simulink model "DinsatHW7"  (R2021b)
settings: Solver=ode45  StartTime=0.0  StopTime=900  RelTol=1e-3
undefined symbols (not defined in the file): IAU
libraries: slpidlib x6, simulink_extras x3, aerolibtransform2 x2, vrlib x1
settings Model: PacingRate=1000  Creator=hilmi  LastModifiedBy=hilmi

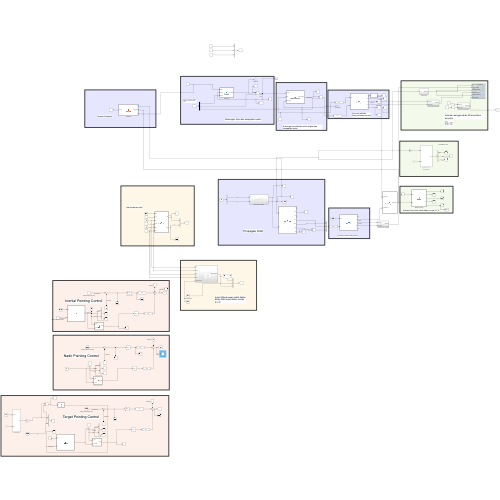
[thumbnail: Simulink's stored preview of the top-level diagram]
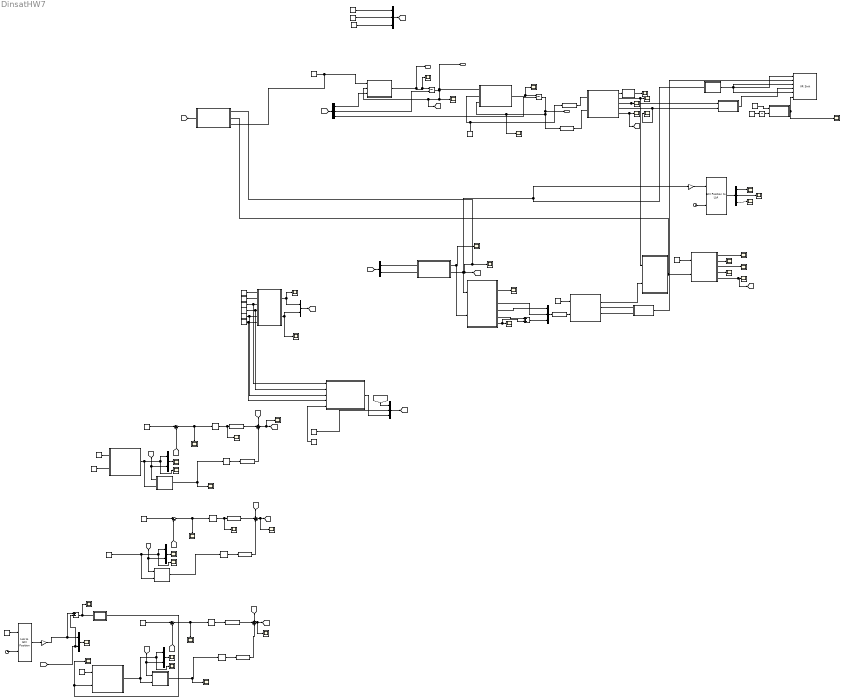
== system DinsatHW7 ==
  note: Gravity Gradient
  note: Inertial Pointing Control
  note: Input elemen orbit
  note: Koordinat LLA
  note: Attitude Body-Orbit satelit dalam urutan Z-Y-X
  note: Input Attitude awal satelit dalam
      | Body-Orbit input dalam urutan
      | Z-Y-X
  note: Koordinat orbit terhadap inersial
  note: Propagasi Orbit
  note: Input Torsi dan initial condition
      | tergantung keperluan setiap
      | nomor.
  note: notes:
      | Sumbu x+ : Merah
      | Sumbu y+ : Biru
      | Sumbu z+ : Hijau
  note: Animasi menggunakan 3D simulation simulink
  note: Konversi attitude
      | Body terhadap inersial
  note: Hubungan perubahan euler angles dan kecepatan sudut
  note: Hubungan torsi dan kecepatan sudut
  note: Nadir Pointing Control
  note: Target Pointing Control
  Add : Sum
  Add1 : Sum  Inputs=+-
  Attitude Body Orbit : MATLAB Function  TreatAsAtomicUnit=on
  BodyOrbit attitude input : Constant  Value=[30,20,30]
  Clock : Clock
  Clock1 : Clock
  Constant{,1,5,25} (4 alike) : Constant  Value=[3,2,1]
  Constant15 : Constant  Value=6903
  Constant19 : Constant  Value=0
  Constant2 : Constant  Value=[1,0,0,0]
  Constant20 : Constant  Value=1e-5
  Constant21 : Constant  Value=1e-4
  Constant22 : Constant  Value=1e-4
  Constant23 : Constant  Value=90
  Constant24 : Constant  Value=[3,1,3]
  Constant26 : Constant  Value=[0,0,1]
  Constant27 : Constant  Value=360/(8.616409000000000e+04)
  Constant4 : Constant  Value=[-7,108,0]
  Constant6 : Constant  Value=[1e-5 1e-5 1e-5]
  Constant7 : Constant  Value=[13.33,-0.087,-0.004;-0.087,13.33,-0.03;-0.04,-0.03,1.33]
  Constant8 : Constant  Value=[1e-5 1e-5 1e-5]
  Constant9 : Constant  Value=[1e-5 1e-5 1e-5]
  Demux : Demux  Outputs=2
  Demux1 : Demux  Outputs=3
  Demux2 : Demux  Outputs=3
  Dynamic Eq : MATLAB Function  TreatAsAtomicUnit=on
  ECI Position to LLA : aerolibtransform2/ECI Position to LLA  red=IAU-2000/2006  year=2024  month=March  day=20  hour=12  min=7  sec=6  deltaT=Sec  errorflag=Error  extraparamflag=off  eunits=Metric (MKS)  earthmodel=WGS84  flat=1/298.257223563  eqradius=6378137
      settings: AttributesFormatString=%<red>  SourceProductBaseCode=AE
  Gain : Gain  Gain=0.001
  Gain2 : Gain  Gain=1000
  GravityGrad : MATLAB Function  TreatAsAtomicUnit=on
  Inertial pointing euler angle : Constant  Value=[0,0,0]
  Inertial pointing euler angle1 : Constant  Value=[0,0,10]
  Inertial pointing euler angle2 : Constant  Value=[0,0,0]
  Inertial pointing euler angle3 : Constant  Value=[0,0,0]
  Integrator : Integrator  InitialConditionSource=external  InitialCondition=[1,3,4]
  Integrator1 : Integrator  InitialConditionSource=external  InitialCondition=[20,30,40]
  Integrator2 : Integrator  InitialCondition=90
  LLA to ECI Position : aerolibtransform2/LLA to ECI Position  red=IAU-2000/2006  year=2024  month=March  day=20  hour=12  min=7  sec=6  deltaT=Sec  errorflag=Error  extraparamflag=off  eunits=Metric (MKS)  earthmodel=WGS84  flat=1/298.257223563  eqradius=6378137
      settings: AttributesFormatString=%<red>  SourceProductBaseCode=AE
  MATLAB Function : MATLAB Function  TreatAsAtomicUnit=on
  MATLAB Function1 : MATLAB Function  TreatAsAtomicUnit=on
  MATLAB Function10 : MATLAB Function  TreatAsAtomicUnit=on
  MATLAB Function12 : MATLAB Function  TreatAsAtomicUnit=on
  MATLAB Function13 : MATLAB Function  TreatAsAtomicUnit=on
  MATLAB Function2 : MATLAB Function  TreatAsAtomicUnit=on
  MATLAB Function3 : MATLAB Function  TreatAsAtomicUnit=on
  MATLAB Function4 : MATLAB Function  TreatAsAtomicUnit=on
  MATLAB Function5 : MATLAB Function  TreatAsAtomicUnit=on
  MATLAB Function6 : MATLAB Function  TreatAsAtomicUnit=on
  MATLAB Function7 : MATLAB Function  TreatAsAtomicUnit=on
  MATLAB Function8 : MATLAB Function  TreatAsAtomicUnit=on
  MATLAB Function9 : MATLAB Function  TreatAsAtomicUnit=on
  Mux{,1,3..4,7} (5 alike) : Mux  Inputs=2
  Mux2 : Mux  Inputs=3
  Mux8 : Mux  Inputs=3
  Mux9 : Mux  Inputs=3
  Newton Gravity Equation : Subsystem
  Omega awal input : Constant  Value=[10,30,40]
  PID Controller1 : slpidlib/PID Controller  Controller=P  Form=Parallel  TimeDomain=Continuous-time  UseExternalTs=off  SampleTime=-1  IntegratorMethod=Forward Euler  FilterMethod=Forward Euler  ControllerParametersSource=internal  P=-6  I=0.001  D=0  UseFilter=on  N=100  TunerSelectOption=Transfer Function Based (PID Tuner App)  InitialConditionSource=internal  InitialConditionForIntegrator=0  InitialConditionForFilter=0  DifferentiatorICPrevScaledInput=0  ExternalReset=none  TrackingMode=off  Kt=1  LimitOutput=off  SatLimitsSource=internal  UpperSaturationLimit=inf  LowerSaturationLimit=-inf  LinearizeAsGain=on  AntiWindupMode=none  Kb=1  POutMin=[]  POutMax=[]  IOutMin=[]  IOutMax=[]  DOutMin=[]  DOutMax=[]  NOutMin=[]  NOutMax=[]  SumOutMin=[]  SumOutMax=[]  SaturationOutMin=[]  SaturationOutMax=[]  PParamMin=[]  PParamMax=[]  IParamMin=[]  IParamMax=[]  DParamMin=[]  DParamMax=[]  NParamMin=[]  NParamMax=[]  KbParamMin=[]  KbParamMax=[]  KtParamMin=[]  KtParamMax=[]  KbOutMin=[]  KbOutMax=[]  KtOutMin=[]  KtOutMax=[]  IntegratorOutMin=[]  IntegratorOutMax=[]  FilterOutMin=[]  FilterOutMax=[]  SumI1OutMin=[]  SumI1OutMax=[]  SumI2OutMin=[]  SumI2OutMax=[]  SumI3OutMin=[]  SumI3OutMax=[]  SumI4OutMin=[]  SumI4OutMax=[]  SumDOutMin=[]  SumDOutMax=[]  DifferentiatorOutMin=[]  DifferentiatorOutMax=[]  FilterDiffOutCoefMin=[]  FilterDiffOutCoefMax=[]  ReciprocalOutMin=[]  ReciprocalOutMax=[]  SumDenOutMin=[]  SumDenOutMax=[]  SumNumOutMin=[]  SumNumOutMax=[]  DivideOutMin=[]  DivideOutMax=[]  UdiffTsProdOutMin=[]  UdiffTsProdOutMax=[]  NTsProdOutMin=[]  NTsProdOutMax=[]  UintegralTsProdOutMin=[]  UintegralTsProdOutMax=[]  UngainTsProdOutMin=[]  UngainTsProdOutMax=[]  IntegratorContinuousStateAttributes=''  IntegratorStateMustResolveToSignalObject=off  IntegratorRTWStateStorageClass=Auto  FilterContinuousStateAttributes=''  FilterStateMustResolveToSignalObject=off  FilterRTWStateStorageClass=Auto  ParallelPVariant=InternalParameters  IdealPVariant=Disabled  IVariant=Disabled  DVariant=Disabled  IntegratorVariant=Disabled  SatVariant=Disabled  AWVariant=Disabled  PCopyVariant=Disabled  TRVariant=Disabled  FdbkBlocksVariant=Forward  IdealPFdbkVariant=Disabled  SatFdbkVariant=Disabled  DerivativeFilterVariant=Disabled  NVariant=Disabled  NCopyVariant=Disabled_SignalSpec  FilterICVariant=Disabled  IntegratorICVariant=Disabled  ExternalResetVariant=Disabled  TRSumVariant=Passthrough  SumFdbkVariant=Disabled  SumVariant=Passthrough_P  TsampFilterVariant=InternalTs  TsampNgainVariant=Passthrough  TsampIntegralVariant=Disabled_SignalSpec  ExternalSaturationOutDataTypeStr=Inherit: Same as second input
  PID Controller2 : slpidlib/PID Controller  Controller=P  Form=Parallel  TimeDomain=Continuous-time  UseExternalTs=off  SampleTime=-1  IntegratorMethod=Forward Euler  FilterMethod=Forward Euler  ControllerParametersSource=internal  P=0.1  I=0.001  D=0  UseFilter=on  N=100  TunerSelectOption=Transfer Function Based (PID Tuner App)  InitialConditionSource=internal  InitialConditionForIntegrator=0  InitialConditionForFilter=0  DifferentiatorICPrevScaledInput=0  ExternalReset=none  TrackingMode=off  Kt=1  LimitOutput=off  SatLimitsSource=internal  UpperSaturationLimit=inf  LowerSaturationLimit=-inf  LinearizeAsGain=on  AntiWindupMode=none  Kb=1  POutMin=[]  POutMax=[]  IOutMin=[]  IOutMax=[]  DOutMin=[]  DOutMax=[]  NOutMin=[]  NOutMax=[]  SumOutMin=[]  SumOutMax=[]  SaturationOutMin=[]  SaturationOutMax=[]  PParamMin=[]  PParamMax=[]  IParamMin=[]  IParamMax=[]  DParamMin=[]  DParamMax=[]  NParamMin=[]  NParamMax=[]  KbParamMin=[]  KbParamMax=[]  KtParamMin=[]  KtParamMax=[]  KbOutMin=[]  KbOutMax=[]  KtOutMin=[]  KtOutMax=[]  IntegratorOutMin=[]  IntegratorOutMax=[]  FilterOutMin=[]  FilterOutMax=[]  SumI1OutMin=[]  SumI1OutMax=[]  SumI2OutMin=[]  SumI2OutMax=[]  SumI3OutMin=[]  SumI3OutMax=[]  SumI4OutMin=[]  SumI4OutMax=[]  SumDOutMin=[]  SumDOutMax=[]  DifferentiatorOutMin=[]  DifferentiatorOutMax=[]  FilterDiffOutCoefMin=[]  FilterDiffOutCoefMax=[]  ReciprocalOutMin=[]  ReciprocalOutMax=[]  SumDenOutMin=[]  SumDenOutMax=[]  SumNumOutMin=[]  SumNumOutMax=[]  DivideOutMin=[]  DivideOutMax=[]  UdiffTsProdOutMin=[]  UdiffTsProdOutMax=[]  NTsProdOutMin=[]  NTsProdOutMax=[]  UintegralTsProdOutMin=[]  UintegralTsProdOutMax=[]  UngainTsProdOutMin=[]  UngainTsProdOutMax=[]  IntegratorContinuousStateAttributes=''  IntegratorStateMustResolveToSignalObject=off  IntegratorRTWStateStorageClass=Auto  FilterContinuousStateAttributes=''  FilterStateMustResolveToSignalObject=off  FilterRTWStateStorageClass=Auto  ParallelPVariant=InternalParameters  IdealPVariant=Disabled  IVariant=Disabled  DVariant=Disabled  IntegratorVariant=Disabled  SatVariant=Disabled  AWVariant=Disabled  PCopyVariant=Disabled  TRVariant=Disabled  FdbkBlocksVariant=Forward  IdealPFdbkVariant=Disabled  SatFdbkVariant=Disabled  DerivativeFilterVariant=Disabled  NVariant=Disabled  NCopyVariant=Disabled_SignalSpec  FilterICVariant=Disabled  IntegratorICVariant=Disabled  ExternalResetVariant=Disabled  TRSumVariant=Passthrough  SumFdbkVariant=Disabled  SumVariant=Passthrough_P  TsampFilterVariant=InternalTs  TsampNgainVariant=Passthrough  TsampIntegralVariant=Disabled_SignalSpec  ExternalSaturationOutDataTypeStr=Inherit: Same as second input
  PID Controller3 : slpidlib/PID Controller  Controller=P  Form=Parallel  TimeDomain=Continuous-time  UseExternalTs=off  SampleTime=-1  IntegratorMethod=Forward Euler  FilterMethod=Forward Euler  ControllerParametersSource=internal  P=-6  I=0.001  D=0  UseFilter=on  N=100  TunerSelectOption=Transfer Function Based (PID Tuner App)  InitialConditionSource=internal  InitialConditionForIntegrator=0  InitialConditionForFilter=0  DifferentiatorICPrevScaledInput=0  ExternalReset=none  TrackingMode=off  Kt=1  LimitOutput=off  SatLimitsSource=internal  UpperSaturationLimit=inf  LowerSaturationLimit=-inf  LinearizeAsGain=on  AntiWindupMode=none  Kb=1  POutMin=[]  POutMax=[]  IOutMin=[]  IOutMax=[]  DOutMin=[]  DOutMax=[]  NOutMin=[]  NOutMax=[]  SumOutMin=[]  SumOutMax=[]  SaturationOutMin=[]  SaturationOutMax=[]  PParamMin=[]  PParamMax=[]  IParamMin=[]  IParamMax=[]  DParamMin=[]  DParamMax=[]  NParamMin=[]  NParamMax=[]  KbParamMin=[]  KbParamMax=[]  KtParamMin=[]  KtParamMax=[]  KbOutMin=[]  KbOutMax=[]  KtOutMin=[]  KtOutMax=[]  IntegratorOutMin=[]  IntegratorOutMax=[]  FilterOutMin=[]  FilterOutMax=[]  SumI1OutMin=[]  SumI1OutMax=[]  SumI2OutMin=[]  SumI2OutMax=[]  SumI3OutMin=[]  SumI3OutMax=[]  SumI4OutMin=[]  SumI4OutMax=[]  SumDOutMin=[]  SumDOutMax=[]  DifferentiatorOutMin=[]  DifferentiatorOutMax=[]  FilterDiffOutCoefMin=[]  FilterDiffOutCoefMax=[]  ReciprocalOutMin=[]  ReciprocalOutMax=[]  SumDenOutMin=[]  SumDenOutMax=[]  SumNumOutMin=[]  SumNumOutMax=[]  DivideOutMin=[]  DivideOutMax=[]  UdiffTsProdOutMin=[]  UdiffTsProdOutMax=[]  NTsProdOutMin=[]  NTsProdOutMax=[]  UintegralTsProdOutMin=[]  UintegralTsProdOutMax=[]  UngainTsProdOutMin=[]  UngainTsProdOutMax=[]  IntegratorContinuousStateAttributes=''  IntegratorStateMustResolveToSignalObject=off  IntegratorRTWStateStorageClass=Auto  FilterContinuousStateAttributes=''  FilterStateMustResolveToSignalObject=off  FilterRTWStateStorageClass=Auto  ParallelPVariant=InternalParameters  IdealPVariant=Disabled  IVariant=Disabled  DVariant=Disabled  IntegratorVariant=Disabled  SatVariant=Disabled  AWVariant=Disabled  PCopyVariant=Disabled  TRVariant=Disabled  FdbkBlocksVariant=Forward  IdealPFdbkVariant=Disabled  SatFdbkVariant=Disabled  DerivativeFilterVariant=Disabled  NVariant=Disabled  NCopyVariant=Disabled_SignalSpec  FilterICVariant=Disabled  IntegratorICVariant=Disabled  ExternalResetVariant=Disabled  TRSumVariant=Passthrough  SumFdbkVariant=Disabled  SumVariant=Passthrough_P  TsampFilterVariant=InternalTs  TsampNgainVariant=Passthrough  TsampIntegralVariant=Disabled_SignalSpec  ExternalSaturationOutDataTypeStr=Inherit: Same as second input
  PID Controller4 : slpidlib/PID Controller  Controller=P  Form=Parallel  TimeDomain=Continuous-time  UseExternalTs=off  SampleTime=-1  IntegratorMethod=Forward Euler  FilterMethod=Forward Euler  ControllerParametersSource=internal  P=0.1  I=0.001  D=0  UseFilter=on  N=100  TunerSelectOption=Transfer Function Based (PID Tuner App)  InitialConditionSource=internal  InitialConditionForIntegrator=0  InitialConditionForFilter=0  DifferentiatorICPrevScaledInput=0  ExternalReset=none  TrackingMode=off  Kt=1  LimitOutput=off  SatLimitsSource=internal  UpperSaturationLimit=inf  LowerSaturationLimit=-inf  LinearizeAsGain=on  AntiWindupMode=none  Kb=1  POutMin=[]  POutMax=[]  IOutMin=[]  IOutMax=[]  DOutMin=[]  DOutMax=[]  NOutMin=[]  NOutMax=[]  SumOutMin=[]  SumOutMax=[]  SaturationOutMin=[]  SaturationOutMax=[]  PParamMin=[]  PParamMax=[]  IParamMin=[]  IParamMax=[]  DParamMin=[]  DParamMax=[]  NParamMin=[]  NParamMax=[]  KbParamMin=[]  KbParamMax=[]  KtParamMin=[]  KtParamMax=[]  KbOutMin=[]  KbOutMax=[]  KtOutMin=[]  KtOutMax=[]  IntegratorOutMin=[]  IntegratorOutMax=[]  FilterOutMin=[]  FilterOutMax=[]  SumI1OutMin=[]  SumI1OutMax=[]  SumI2OutMin=[]  SumI2OutMax=[]  SumI3OutMin=[]  SumI3OutMax=[]  SumI4OutMin=[]  SumI4OutMax=[]  SumDOutMin=[]  SumDOutMax=[]  DifferentiatorOutMin=[]  DifferentiatorOutMax=[]  FilterDiffOutCoefMin=[]  FilterDiffOutCoefMax=[]  ReciprocalOutMin=[]  ReciprocalOutMax=[]  SumDenOutMin=[]  SumDenOutMax=[]  SumNumOutMin=[]  SumNumOutMax=[]  DivideOutMin=[]  DivideOutMax=[]  UdiffTsProdOutMin=[]  UdiffTsProdOutMax=[]  NTsProdOutMin=[]  NTsProdOutMax=[]  UintegralTsProdOutMin=[]  UintegralTsProdOutMax=[]  UngainTsProdOutMin=[]  UngainTsProdOutMax=[]  IntegratorContinuousStateAttributes=''  IntegratorStateMustResolveToSignalObject=off  IntegratorRTWStateStorageClass=Auto  FilterContinuousStateAttributes=''  FilterStateMustResolveToSignalObject=off  FilterRTWStateStorageClass=Auto  ParallelPVariant=InternalParameters  IdealPVariant=Disabled  IVariant=Disabled  DVariant=Disabled  IntegratorVariant=Disabled  SatVariant=Disabled  AWVariant=Disabled  PCopyVariant=Disabled  TRVariant=Disabled  FdbkBlocksVariant=Forward  IdealPFdbkVariant=Disabled  SatFdbkVariant=Disabled  DerivativeFilterVariant=Disabled  NVariant=Disabled  NCopyVariant=Disabled_SignalSpec  FilterICVariant=Disabled  IntegratorICVariant=Disabled  ExternalResetVariant=Disabled  TRSumVariant=Passthrough  SumFdbkVariant=Disabled  SumVariant=Passthrough_P  TsampFilterVariant=InternalTs  TsampNgainVariant=Passthrough  TsampIntegralVariant=Disabled_SignalSpec  ExternalSaturationOutDataTypeStr=Inherit: Same as second input
  PID Controller5 : slpidlib/PID Controller  Controller=P  Form=Parallel  TimeDomain=Continuous-time  UseExternalTs=off  SampleTime=-1  IntegratorMethod=Forward Euler  FilterMethod=Forward Euler  ControllerParametersSource=internal  P=-6  I=0.001  D=0  UseFilter=on  N=100  TunerSelectOption=Transfer Function Based (PID Tuner App)  InitialConditionSource=internal  InitialConditionForIntegrator=0  InitialConditionForFilter=0  DifferentiatorICPrevScaledInput=0  ExternalReset=none  TrackingMode=off  Kt=1  LimitOutput=off  SatLimitsSource=internal  UpperSaturationLimit=inf  LowerSaturationLimit=-inf  LinearizeAsGain=on  AntiWindupMode=none  Kb=1  POutMin=[]  POutMax=[]  IOutMin=[]  IOutMax=[]  DOutMin=[]  DOutMax=[]  NOutMin=[]  NOutMax=[]  SumOutMin=[]  SumOutMax=[]  SaturationOutMin=[]  SaturationOutMax=[]  PParamMin=[]  PParamMax=[]  IParamMin=[]  IParamMax=[]  DParamMin=[]  DParamMax=[]  NParamMin=[]  NParamMax=[]  KbParamMin=[]  KbParamMax=[]  KtParamMin=[]  KtParamMax=[]  KbOutMin=[]  KbOutMax=[]  KtOutMin=[]  KtOutMax=[]  IntegratorOutMin=[]  IntegratorOutMax=[]  FilterOutMin=[]  FilterOutMax=[]  SumI1OutMin=[]  SumI1OutMax=[]  SumI2OutMin=[]  SumI2OutMax=[]  SumI3OutMin=[]  SumI3OutMax=[]  SumI4OutMin=[]  SumI4OutMax=[]  SumDOutMin=[]  SumDOutMax=[]  DifferentiatorOutMin=[]  DifferentiatorOutMax=[]  FilterDiffOutCoefMin=[]  FilterDiffOutCoefMax=[]  ReciprocalOutMin=[]  ReciprocalOutMax=[]  SumDenOutMin=[]  SumDenOutMax=[]  SumNumOutMin=[]  SumNumOutMax=[]  DivideOutMin=[]  DivideOutMax=[]  UdiffTsProdOutMin=[]  UdiffTsProdOutMax=[]  NTsProdOutMin=[]  NTsProdOutMax=[]  UintegralTsProdOutMin=[]  UintegralTsProdOutMax=[]  UngainTsProdOutMin=[]  UngainTsProdOutMax=[]  IntegratorContinuousStateAttributes=''  IntegratorStateMustResolveToSignalObject=off  IntegratorRTWStateStorageClass=Auto  FilterContinuousStateAttributes=''  FilterStateMustResolveToSignalObject=off  FilterRTWStateStorageClass=Auto  ParallelPVariant=InternalParameters  IdealPVariant=Disabled  IVariant=Disabled  DVariant=Disabled  IntegratorVariant=Disabled  SatVariant=Disabled  AWVariant=Disabled  PCopyVariant=Disabled  TRVariant=Disabled  FdbkBlocksVariant=Forward  IdealPFdbkVariant=Disabled  SatFdbkVariant=Disabled  DerivativeFilterVariant=Disabled  NVariant=Disabled  NCopyVariant=Disabled_SignalSpec  FilterICVariant=Disabled  IntegratorICVariant=Disabled  ExternalResetVariant=Disabled  TRSumVariant=Passthrough  SumFdbkVariant=Disabled  SumVariant=Passthrough_P  TsampFilterVariant=InternalTs  TsampNgainVariant=Passthrough  TsampIntegralVariant=Disabled_SignalSpec  ExternalSaturationOutDataTypeStr=Inherit: Same as second input
  PID Controller6 : slpidlib/PID Controller  Controller=P  Form=Parallel  TimeDomain=Continuous-time  UseExternalTs=off  SampleTime=-1  IntegratorMethod=Forward Euler  FilterMethod=Forward Euler  ControllerParametersSource=internal  P=0.1  I=0.001  D=0  UseFilter=on  N=100  TunerSelectOption=Transfer Function Based (PID Tuner App)  InitialConditionSource=internal  InitialConditionForIntegrator=0  InitialConditionForFilter=0  DifferentiatorICPrevScaledInput=0  ExternalReset=none  TrackingMode=off  Kt=1  LimitOutput=off  SatLimitsSource=internal  UpperSaturationLimit=inf  LowerSaturationLimit=-inf  LinearizeAsGain=on  AntiWindupMode=none  Kb=1  POutMin=[]  POutMax=[]  IOutMin=[]  IOutMax=[]  DOutMin=[]  DOutMax=[]  NOutMin=[]  NOutMax=[]  SumOutMin=[]  SumOutMax=[]  SaturationOutMin=[]  SaturationOutMax=[]  PParamMin=[]  PParamMax=[]  IParamMin=[]  IParamMax=[]  DParamMin=[]  DParamMax=[]  NParamMin=[]  NParamMax=[]  KbParamMin=[]  KbParamMax=[]  KtParamMin=[]  KtParamMax=[]  KbOutMin=[]  KbOutMax=[]  KtOutMin=[]  KtOutMax=[]  IntegratorOutMin=[]  IntegratorOutMax=[]  FilterOutMin=[]  FilterOutMax=[]  SumI1OutMin=[]  SumI1OutMax=[]  SumI2OutMin=[]  SumI2OutMax=[]  SumI3OutMin=[]  SumI3OutMax=[]  SumI4OutMin=[]  SumI4OutMax=[]  SumDOutMin=[]  SumDOutMax=[]  DifferentiatorOutMin=[]  DifferentiatorOutMax=[]  FilterDiffOutCoefMin=[]  FilterDiffOutCoefMax=[]  ReciprocalOutMin=[]  ReciprocalOutMax=[]  SumDenOutMin=[]  SumDenOutMax=[]  SumNumOutMin=[]  SumNumOutMax=[]  DivideOutMin=[]  DivideOutMax=[]  UdiffTsProdOutMin=[]  UdiffTsProdOutMax=[]  NTsProdOutMin=[]  NTsProdOutMax=[]  UintegralTsProdOutMin=[]  UintegralTsProdOutMax=[]  UngainTsProdOutMin=[]  UngainTsProdOutMax=[]  IntegratorContinuousStateAttributes=''  IntegratorStateMustResolveToSignalObject=off  IntegratorRTWStateStorageClass=Auto  FilterContinuousStateAttributes=''  FilterStateMustResolveToSignalObject=off  FilterRTWStateStorageClass=Auto  ParallelPVariant=InternalParameters  IdealPVariant=Disabled  IVariant=Disabled  DVariant=Disabled  IntegratorVariant=Disabled  SatVariant=Disabled  AWVariant=Disabled  PCopyVariant=Disabled  TRVariant=Disabled  FdbkBlocksVariant=Forward  IdealPFdbkVariant=Disabled  SatFdbkVariant=Disabled  DerivativeFilterVariant=Disabled  NVariant=Disabled  NCopyVariant=Disabled_SignalSpec  FilterICVariant=Disabled  IntegratorICVariant=Disabled  ExternalResetVariant=Disabled  TRSumVariant=Passthrough  SumFdbkVariant=Disabled  SumVariant=Passthrough_P  TsampFilterVariant=InternalTs  TsampNgainVariant=Passthrough  TsampIntegralVariant=Disabled_SignalSpec  ExternalSaturationOutDataTypeStr=Inherit: Same as second input
  Scope{,1..42} (43 alike) : Scope
  Signal Specification{,1,3..8} (8 alike) : SignalSpecification  Dimensions=3
  Signal Specification2 : SignalSpecification  Dimensions=[1 3]
  Subsystem1 : Subsystem
  Sum : Sum  Inputs=+++
  Sum1 : Sum  Inputs=|+-
  Sum2 : Sum  Inputs=+++
  Sum3 : Sum  Inputs=|+-
  Sum4 : Sum  Inputs=+++
  Sum5 : Sum  Inputs=|+-
  Transformasi ke 3D World : Subsystem
  Transformasi ke 3D World1 : Subsystem
  Transformasi ke 3D World2 : Subsystem
  Ubah sumbu : Subsystem
  VR Sink1 : vrlib/VR Sink  InstantiateOnLoad=on  SampleTime=0.1  ViewEnable=on  RemoteChange=off  RemoteView=off  FieldsWritten=CameraRear.translation.3.1.1.double#Orbital.rotation.4.1.1.double#Orbital.translation.3.1.1.double#Satellite.rotation.4.1.1.double#Satellite.translation.3.1.1.double#Earth.rotation.4.1.1.double  WorldFileName=satwithaxis.x3d  WorldDescription=Satellite Vehicle  AutoView=off  VideoDimensions=[]  AllowVariableSize=off
  omegaDot : Outport
  EulerAngles : Outport  Port=2
  omega : Outport  Port=3
  wires:
  Dynamic Eq/1(omegaDot) -> omegaDot/1, Scope7/1, Integrator/1  "omegaDot"
  Integrator/1 -> omega/1, MATLAB Function/1(omega), [Omega], Dynamic Eq/2(omega), Scope1/1  "omega"
  Constant1/1 -> MATLAB Function/2(seq), Signal Specification1/1
  Integrator1/1 -> EulerAngles/1, Scope/1, MATLAB Function/3(EulerAngle), Signal Specification/1  "EulerAngles"
  Constant7/1 -> GravityGrad/3(I), Dynamic Eq/1(Inertia)
  MATLAB Function/1(EulerAngleDot) -> Scope8/1, Integrator1/1  "EulerAngleDot"
  MATLAB Function1/5(q) -> [Inertialq], Scope2/1  "Quaternion"
  Signal Specification/1 -> MATLAB Function1/2("t ")
  Signal Specification1/1 -> MATLAB Function1/1(seq)
  MATLAB Function1/4(ph) -> Transformasi ke 3D World/2(EulerAngle), Scope3/1  "EulerAngle"
  MATLAB Function1/3(a) -> Transformasi ke 3D World/1(EulerAxis), Scope4/1  "EulerAxis"
  MATLAB Function1/2(R) -> MATLAB Function6/1(R_BodyIner), Scope5/1  "RotMat"
  Constant6/1 -> Mux2/1
  [InputBodyOrbit] -> Demux1/1
  Demux1/1 -> Dynamic Eq/3(Torsion)
  Demux1/2 -> Integrator/2
  Demux1/3 -> Integrator1/2
  Mux2/1 -> [TesNormal]
  Constant8/1 -> Mux2/2
  Constant9/1 -> Mux2/3
  MATLAB Function2/1(t) -> Scope6/1  "EulerAngles"
  [InputKepler] -> Demux/1
  Demux/1 -> Newton Gravity Equation/1(v0)  "v0"
  Demux/2 -> Newton Gravity Equation/2(r0)  "r0"
  Newton Gravity Equation/1(v) -> MATLAB Function4/2(v), Scope14/1
  Newton Gravity Equation/2(r) -> Ubah sumbu/1(r), Gain2/1, MATLAB Function4/1(r), [OrbitR], GravityGrad/1(r), Scope13/1
  Mux7/1 -> [InputKepler]
  MATLAB Function3/1(v_init) -> Mux7/1, Scope16/1  "v_init"
  MATLAB Function3/2(r_init) -> Mux7/2, Scope17/1  "r_init"
  Constant19/1 -> MATLAB Function3/2(ecc)
  Constant15/1 -> MATLAB Function3/1(sma)
  MATLAB Function4/7(TA) -> Add/2, Scope15/1
  Constant24/1 -> MATLAB Function5/1(seq)
  MATLAB Function4/5(node) -> Mux8/1
  MATLAB Function4/4(inc) -> Mux8/2
  MATLAB Function4/6(aop) -> Add/1
  Add/1 -> Mux8/3
  Mux8/1 -> Signal Specification2/1
  Signal Specification2/1 -> MATLAB Function5/2("t ")
  MATLAB Function6/1(RBodyOrbit) -> GravityGrad/2(R_bodyorb), Attitude Body Orbit/2("R ")
  MATLAB Function5/2(R) -> MATLAB Function6/2(R_OrbitInertial)  "RotMat"
  Constant25/1 -> Attitude Body Orbit/1(seq)
  MATLAB Function5/3(a) -> Transformasi ke 3D World1/1(EulerAxis)  "EulerAxis"
  MATLAB Function5/4(ph) -> Transformasi ke 3D World1/2(EulerAngle)  "EulerAngle"
  Ubah sumbu/1(Translation) -> VR Sink1/5, VR Sink1/1, VR Sink1/3
  Transformasi ke 3D World1/1(StateOut) -> VR Sink1/2
  Transformasi ke 3D World/1(StateOut) -> VR Sink1/4
  Integrator2/1 -> Transformasi ke 3D World2/2(EulerAngle)
  Constant26/1 -> Transformasi ke 3D World2/1(EulerAxis)
  Constant27/1 -> Integrator2/1
  Transformasi ke 3D World2/1(StateOut) -> VR Sink1/6, Scope18/1
  Constant23/1 -> Subsystem1/4(TA), MATLAB Function3/6(TA)
  Constant22/1 -> Subsystem1/3(aop), MATLAB Function3/5(aop)
  Constant20/1 -> Subsystem1/1(inc), MATLAB Function3/3(inc)
  Constant21/1 -> Subsystem1/2(node), MATLAB Function3/4(node)
  BodyOrbit attitude input/1 -> Subsystem1/5(BodyOrbitInput)
  Omega awal input/1 -> Mux9/2
  Subsystem1/1(BodyInertialInput) -> Mux9/3
  Mux9/1 -> [InputBodyOrbit]
  Attitude Body Orbit/1(t) -> Scope19/1
  Attitude Body Orbit/2(R) -> Scope20/1
  Attitude Body Orbit/3(a) -> Scope21/1
  Attitude Body Orbit/4(ph) -> Scope22/1
  Attitude Body Orbit/5(q) -> [Orbitq], Scope23/1
  Clock/1 -> ECI Position to LLA/2
  ECI Position to LLA/1 -> Demux2/1
  Demux2/1 -> Scope24/1  "Lintang"
  Demux2/2 -> Scope25/1  "Bujur"
  Demux2/3 -> Scope26/1  "Tinggi"
  Gain2/1 -> ECI Position to LLA/1
  MATLAB Function4/2(sma) -> Scope27/1
  GravityGrad/1(Torsion) -> [GravityGrad]
  [GravityGrad] -> Sum/1
  Inertial pointing euler angle/1 -> Sum1/1  "DesiredInertial"
  [Omega] -> Sum1/2  "InertialEuler"
  PID Controller2/1 -> Scope10/1, Signal Specification3/1
  MATLAB Function1/1(t) -> MATLAB Function2/1(u)
  Sum1/1 -> Scope12/1, PID Controller2/1
  Signal Specification3/1 -> Sum/2
  Signal Specification4/1 -> Sum/3
  Inertial pointing euler angle1/1 -> MATLAB Function9/2(t)  "DesiredInertial"
  PID Controller1/1 -> Signal Specification4/1
  Constant/1 -> MATLAB Function9/1(seq)
  MATLAB Function9/1(q) -> Scope30/1, Mux/1, MATLAB Function8/2(q_comm)  "q_desired"
  [Inertialq] -> MATLAB Function8/1(q_real), Mux/2  "q_real"
  MATLAB Function8/1(sigma) -> Scope29/1, PID Controller1/1
  Mux/1 -> Scope28/1
  Constant2/1 -> Scope35/1, Mux1/1, MATLAB Function7/2(q_comm)  "q_desired"
  PID Controller3/1 -> Signal Specification6/1
  Signal Specification5/1 -> Sum2/2
  Mux1/1 -> Scope33/1
  [GravityGrad] -> Sum2/1
  Inertial pointing euler angle2/1 -> Sum3/1  "DesiredInertial"
  MATLAB Function7/1(sigma) -> PID Controller3/1
  Signal Specification6/1 -> Sum2/3
  [Orbitq] -> MATLAB Function7/1(q_real), Mux1/2  "q_real"
  [Omega] -> Sum3/2  "InertialEuler"
  Sum3/1 -> Scope32/1, PID Controller4/1
  PID Controller4/1 -> Scope31/1, Signal Specification5/1
  Sum/1 -> Scope11/1, [InertialPointing]  "Moment"
  [NadirPointing] -> Mux9/1
  Sum2/1 -> Scope34/1, [NadirPointing]  "Moment"
  Sum4/1 -> Scope36/1, [TargetPointing]  "Moment"
  PID Controller6/1 -> Signal Specification7/1
  Signal Specification8/1 -> Sum4/3
  MATLAB Function10/1(sigma) -> Scope39/1, PID Controller5/1
  [Inertialq] -> MATLAB Function10/1(q_real), Mux3/2  "q_real"
  Sum5/1 -> Scope37/1, PID Controller6/1
  [GravityGrad] -> Sum4/1
  Inertial pointing euler angle3/1 -> Sum5/1  "DesiredInertial"
  Signal Specification7/1 -> Sum4/2
  [Omega] -> Sum5/2  "InertialEuler"
  Mux3/1 -> Scope38/1
  MATLAB Function12/1(q) -> Scope40/1, Mux3/1, MATLAB Function10/2(q_comm)  "q_desired"
  PID Controller5/1 -> Signal Specification8/1
  Clock1/1 -> LLA to ECI Position/2
  Constant4/1 -> LLA to ECI Position/1
  LLA to ECI Position/1 -> Gain/1
  Gain/1 -> Add1/1, Mux4/1  "X"
  [OrbitR] -> Add1/2, Mux4/2  "R"
  Constant5/1 -> MATLAB Function12/1(seq)
  MATLAB Function13/1(y) -> Scope42/1, MATLAB Function12/2(t)  "DesiredInertial"
  Mux4/1 -> Scope41/1
  Add1/1 -> MATLAB Function13/1(u), Scope9/1

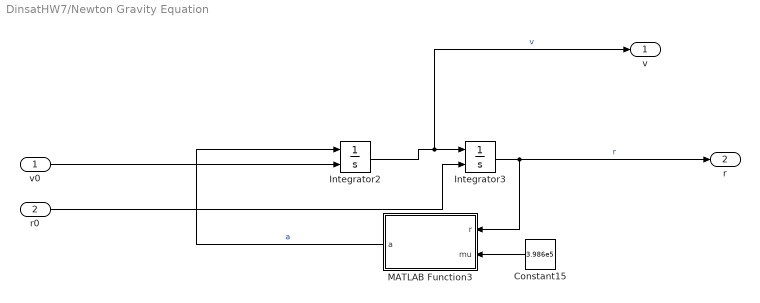
== system DinsatHW7/Newton Gravity Equation ==
  v0 : Inport
  r0 : Inport  Port=2
  Constant15 : Constant  Value=3.986e5
  Integrator2 : Integrator  InitialConditionSource=external
  Integrator3 : Integrator  InitialConditionSource=external
  MATLAB Function3 : MATLAB Function  TreatAsAtomicUnit=on
  v : Outport
  r : Outport  Port=2
  wires:
  Integrator3/1 -> r/1, MATLAB Function3/1(r)  "r"
  r0/1 -> Integrator3/2
  Integrator2/1 -> v/1, Integrator3/1  "v"
  MATLAB Function3/1(a) -> Integrator2/1  "a"
  Constant15/1 -> MATLAB Function3/2(mu)
  v0/1 -> Integrator2/2

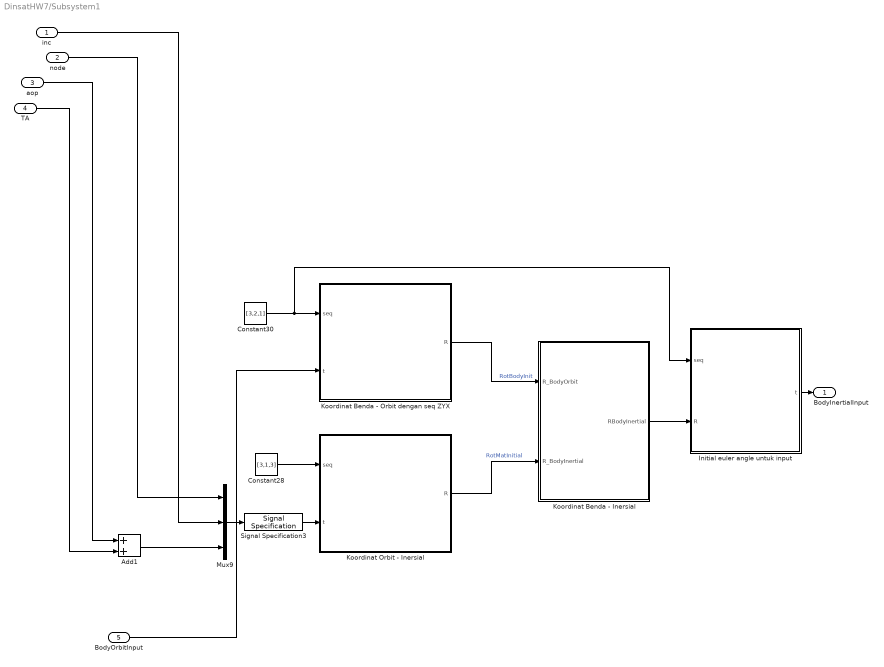
== system DinsatHW7/Subsystem1 ==
  inc : Inport
  node : Inport  Port=2
  aop : Inport  Port=3
  TA : Inport  Port=4
  BodyOrbitInput : Inport  Port=5
  Add1 : Sum
  Constant28 : Constant  Value=[3,1,3]
  Constant30 : Constant  Value=[3,2,1]
  Initial euler angle untuk input : MATLAB Function  TreatAsAtomicUnit=on
  Koordinat Benda - Inersial : MATLAB Function  TreatAsAtomicUnit=on
  Koordinat Benda - Orbit dengan seq ZYX : MATLAB Function  TreatAsAtomicUnit=on
  Koordinat Orbit - Inersial : MATLAB Function  TreatAsAtomicUnit=on
  Mux9 : Mux  Inputs=3
  Signal Specification3 : SignalSpecification  Dimensions=[1 3]
  BodyInertialInput : Outport
  wires:
  Signal Specification3/1 -> Koordinat Orbit - Inersial/2(t)
  Constant30/1 -> Initial euler angle untuk input/1(seq), Koordinat Benda - Orbit dengan seq ZYX/1(seq)
  Mux9/1 -> Signal Specification3/1
  aop/1 -> Add1/1
  BodyOrbitInput/1 -> Koordinat Benda - Orbit dengan seq ZYX/2(t)
  Add1/1 -> Mux9/3
  Constant28/1 -> Koordinat Orbit - Inersial/1(seq)
  Koordinat Benda - Inersial/1(RBodyInertial) -> Initial euler angle untuk input/2(R)
  Koordinat Orbit - Inersial/1(R) -> Koordinat Benda - Inersial/2(R_BodyInertial)  "RotMatInitial"
  Koordinat Benda - Orbit dengan seq ZYX/1(R) -> Koordinat Benda - Inersial/1(R_BodyOrbit)  "RotBodyInit"
  Initial euler angle untuk input/1(t) -> BodyInertialInput/1
  inc/1 -> Mux9/2
  TA/1 -> Add1/2
  node/1 -> Mux9/1

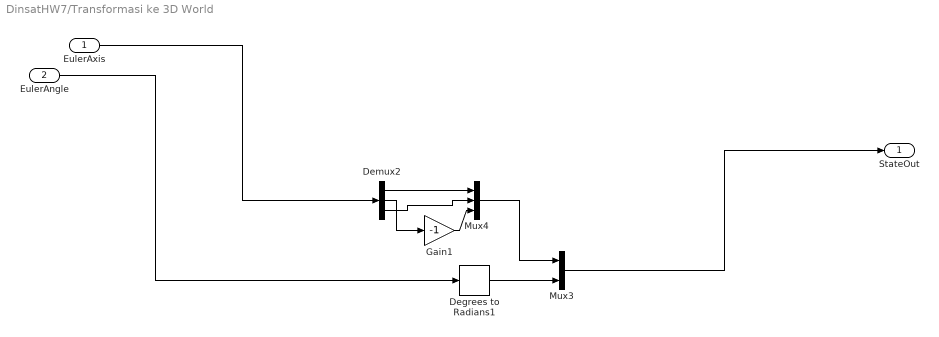
== system DinsatHW7/Transformasi ke 3D World ==
  EulerAxis : Inport
  EulerAngle : Inport  Port=2
  Degrees to Radians1 : simulink_extras/Transformations/Degrees to Radians
  Demux2 : Demux  Outputs=3
  Gain1 : Gain  Gain=-1
  Mux3 : Mux  Inputs=2
  Mux4 : Mux  Inputs=3
  StateOut : Outport
  wires:
  Mux3/1 -> StateOut/1
  Degrees to Radians1/1 -> Mux3/2
  Demux2/3 -> Mux4/2
  EulerAngle/1 -> Degrees to Radians1/1
  Demux2/1 -> Mux4/1
  EulerAxis/1 -> Demux2/1
  Demux2/2 -> Gain1/1
  Mux4/1 -> Mux3/1
  Gain1/1 -> Mux4/3

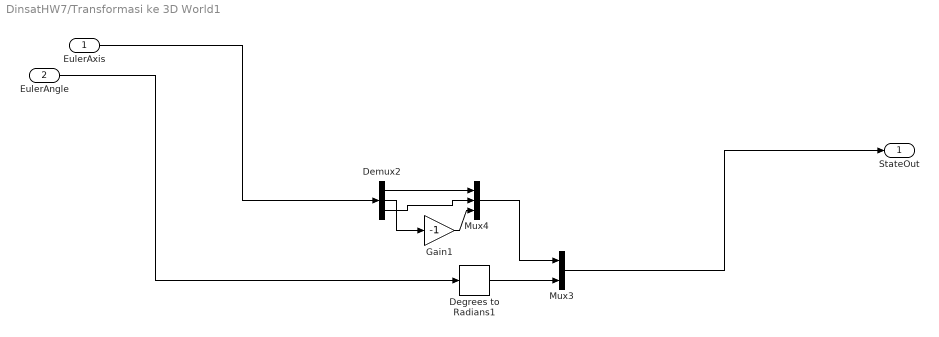
== system DinsatHW7/Transformasi ke 3D World1 ==
  EulerAxis : Inport
  EulerAngle : Inport  Port=2
  Degrees to Radians1 : simulink_extras/Transformations/Degrees to Radians
  Demux2 : Demux  Outputs=3
  Gain1 : Gain  Gain=-1
  Mux3 : Mux  Inputs=2
  Mux4 : Mux  Inputs=3
  StateOut : Outport
  wires:
  Mux3/1 -> StateOut/1
  Degrees to Radians1/1 -> Mux3/2
  Demux2/3 -> Mux4/2
  EulerAngle/1 -> Degrees to Radians1/1
  Demux2/1 -> Mux4/1
  EulerAxis/1 -> Demux2/1
  Demux2/2 -> Gain1/1
  Mux4/1 -> Mux3/1
  Gain1/1 -> Mux4/3

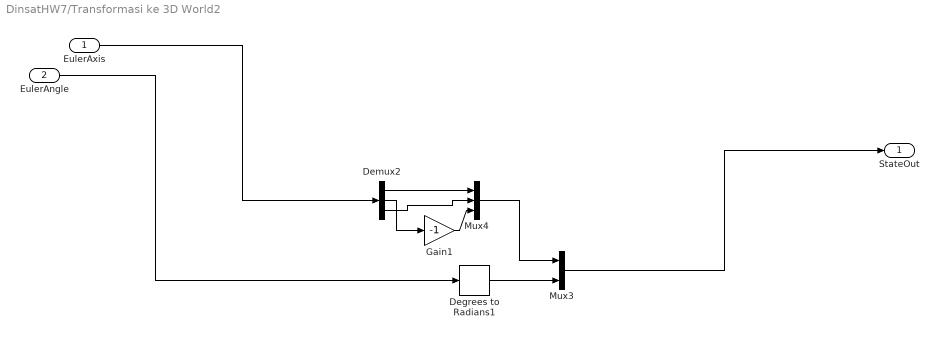
== system DinsatHW7/Transformasi ke 3D World2 ==
  EulerAxis : Inport
  EulerAngle : Inport  Port=2
  Degrees to Radians1 : simulink_extras/Transformations/Degrees to Radians
  Demux2 : Demux  Outputs=3
  Gain1 : Gain  Gain=-1
  Mux3 : Mux  Inputs=2
  Mux4 : Mux  Inputs=3
  StateOut : Outport
  wires:
  Mux3/1 -> StateOut/1
  Degrees to Radians1/1 -> Mux3/2
  Demux2/3 -> Mux4/2
  EulerAngle/1 -> Degrees to Radians1/1
  Demux2/1 -> Mux4/1
  EulerAxis/1 -> Demux2/1
  Demux2/2 -> Gain1/1
  Mux4/1 -> Mux3/1
  Gain1/1 -> Mux4/3

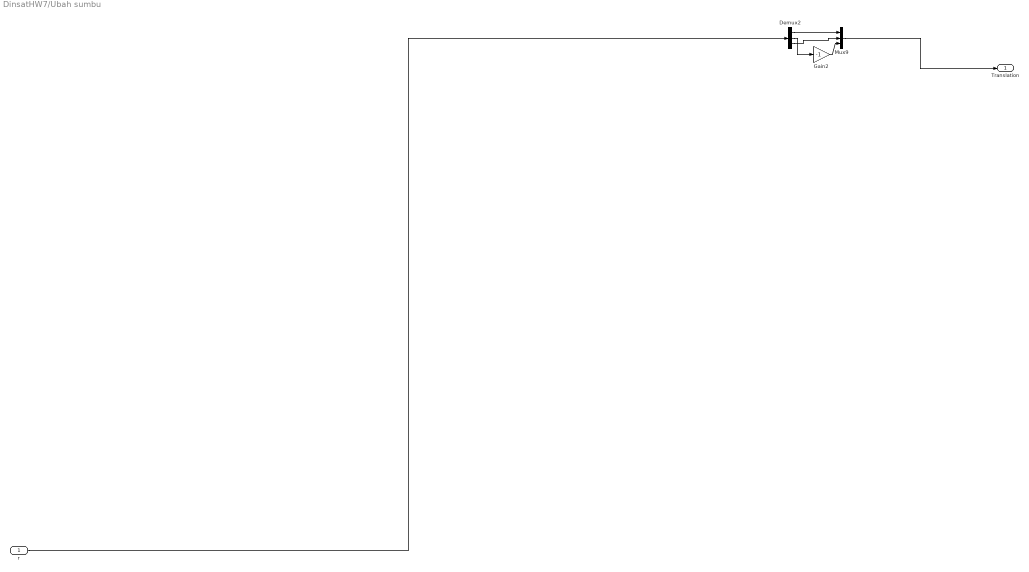
== system DinsatHW7/Ubah sumbu ==
  r : Inport
  Demux2 : Demux  Outputs=3
  Gain2 : Gain  Gain=-1
  Mux9 : Mux  Inputs=3
  Translation : Outport
  wires:
  Gain2/1 -> Mux9/3
  Demux2/1 -> Mux9/1
  Demux2/2 -> Gain2/1
  Demux2/3 -> Mux9/2
  r/1 -> Demux2/1
  Mux9/1 -> Translation/1

== matlab function DinsatHW7/Subsystem1/Koordinat Orbit - Inersial ==
  data: seq input; t input; R output size=[3 3]
function R =EulerAngles(seq,t)
t=deg2rad(t);

%% Rotation Matrix
%Rotasi pertama
i=[mod(seq(1)+1,3),mod(seq(1)+2,3)];
for j=1:2
    if i(j)==0
        i(j)=3;
    end
end
R_1=zeros(3,3);
R_1(i,i)=[cos(t(1)) sin(t(1));-sin(t(1)) cos(t(1))];
R_1(seq(1),seq(1))=1;

%Rotasi kedua
i=[mod(seq(2)+1,3),mod(seq(2)+2,3)];
for j=1:2
    if i(j)==0
        i(j)=3;
    end
end
R_2=zeros(3,3);
R_2(i,i)=[cos(t(2)) sin(t(2));-sin(t(2)) cos(t(2))];
R_2(seq(2),seq(2))=1;

%Rotasi ketiga
i=[mod(seq(3)+1,3),mod(seq(3)+2,3)];
for j=1:2
    if i(j)==0
        i(j)=3;
    end
end
R_3=zeros(3,3);
R_3(i,i)=[cos(t(3)) sin(t(3));-sin(t(3)) cos(t(3))];
R_3(seq(3),seq(3))=1;

% perlu dikali rotasi dua kali lagi supaya benar koordinat orbitalnya
R=[1 0 0;0 0 -1;0 1 0]*[0 1 0;-1 0 0;0 0 1]*R_3*R_2*R_1;

end

== matlab function DinsatHW7/Subsystem1/Koordinat Benda - Orbit dengan seq ZYX ==
  data: seq input; t input; R output size=[3 3]
function R =EulerAngles(seq,t)
t=deg2rad(t);

%% Rotation Matrix
%Rotasi pertama
i=[mod(seq(1)+1,3),mod(seq(1)+2,3)];
for j=1:2
    if i(j)==0
        i(j)=3;
    end
end
R_1=zeros(3,3);
R_1(i,i)=[cos(t(1)) sin(t(1));-sin(t(1)) cos(t(1))];
R_1(seq(1),seq(1))=1;

%Rotasi kedua
i=[mod(seq(2)+1,3),mod(seq(2)+2,3)];
for j=1:2
    if i(j)==0
        i(j)=3;
    end
end
R_2=zeros(3,3);
R_2(i,i)=[cos(t(2)) sin(t(2));-sin(t(2)) cos(t(2))];
R_2(seq(2),seq(2))=1;

%Rotasi ketiga
i=[mod(seq(3)+1,3),mod(seq(3)+2,3)];
for j=1:2
    if i(j)==0
        i(j)=3;
    end
end
R_3=zeros(3,3);
R_3(i,i)=[cos(t(3)) sin(t(3));-sin(t(3)) cos(t(3))];
R_3(seq(3),seq(3))=1;


R=R_3*R_2*R_1;
end

== matlab function DinsatHW7/Subsystem1/Koordinat Benda - Inersial ==
  data: R_BodyOrbit input size=[3 3]; RBodyInertial output size=[3 3]; R_BodyInertial input size=[3 3]
function RBodyInertial = RotMatBodyInertial(R_BodyOrbit, R_BodyInertial)
RBodyInertial=R_BodyOrbit*R_BodyInertial;
end

== matlab function DinsatHW7/Subsystem1/Initial euler angle untuk input ==
  data: seq input size=[1 3]; t output size=[1 3]; R input size=[3 3]
function t =RotMatrix(seq,R)
t1=[0,0];t2=[0,0];t3=[0,0];
notseq=0;
%% Euler angle
if seq(1,1)==seq(1,3)
    t2(1)=acos(R(seq(1),seq(3)));
    t2(2)=-1*t2(1);
    for i=1:3
        if and(seq(1)~=i,seq(2)~=i)
            notseq=i;
        end
    end
    if mod(seq(2)-seq(1),3)==2
    t1=atan2(R(seq(1),seq(2))./sin(t2),R(seq(1),notseq)./sin(t2));
    t3=atan2(R(seq(2),seq(1))./sin(t2),-R(notseq,seq(1))./sin(t2));
    else
    t1=atan2(R(seq(1),seq(2))./sin(t2),-R(seq(1),notseq)./sin(t2));   
    t3=atan2(R(seq(2),seq(1))./sin(t2),R(notseq,seq(1))./sin(t2));
    end
else
    if mod(seq(2)-seq(1),3)==2
    t2(1)=asin(-R(seq(3),seq(1)));
    t2(2)=pi-t2(1);
    t1=atan2(R(seq(3),seq(2))./cos(t2),R(seq(3),seq(3))./cos(t2));
    t3=atan2(R(seq(2),seq(1))./cos(t2),R(seq(1),seq(1))./cos(t2));
    else
    t2(1)=asin(R(seq(3),seq(1)));
    t2(2)=pi-t2(1);
    t1=atan2(-R(seq(3),seq(2))./cos(t2),R(seq(3),seq(3))./cos(t2));
    t3=atan2(-R(seq(2),seq(1))./cos(t2),R(seq(1),seq(1))./cos(t2));
    end   
end

t=[t1(1) t2(1) t3(1)];
t=rad2deg(t);
end

== matlab function DinsatHW7/MATLAB Function1 ==
  data: seq input; t output; t input; R output size=[3 3]; a output size=[3 1]; ph output; q output size=[1 4]
function [t,R,a,ph,q]=EulerAngles(seq,t)
t=deg2rad(t);

%% Rotation Matrix
%Rotasi pertama
i=[mod(seq(1)+1,3),mod(seq(1)+2,3)];
for j=1:2
    if i(j)==0
        i(j)=3;
    end
end
R_1=zeros(3,3);
R_1(i,i)=[cos(t(1)) sin(t(1));-sin(t(1)) cos(t(1))];
R_1(seq(1),seq(1))=1;

%Rotasi kedua
i=[mod(seq(2)+1,3),mod(seq(2)+2,3)];
for j=1:2
    if i(j)==0
        i(j)=3;
    end
end
R_2=zeros(3,3);
R_2(i,i)=[cos(t(2)) sin(t(2));-sin(t(2)) cos(t(2))];
R_2(seq(2),seq(2))=1;

%Rotasi ketiga
i=[mod(seq(3)+1,3),mod(seq(3)+2,3)];
for j=1:2
    if i(j)==0
        i(j)=3;
    end
end
R_3=zeros(3,3);
R_3(i,i)=[cos(t(3)) sin(t(3));-sin(t(3)) cos(t(3))];
R_3(seq(3),seq(3))=1;


R=R_3*R_2*R_1;
%% Euler axis and angle
%euler angle
ph=acos((trace(R)-1)/2);
if or(ph==pi,ph==0)
    a=0.5/sin(ph-1e-5)*([R(2,3)-R(3,2);R(3,1)-R(1,3);R(1,2)-R(2,1)]);
else
    a=0.5/sin(ph)*([R(2,3)-R(3,2);R(3,1)-R(1,3);R(1,2)-R(2,1)]);
end
%% quaternion
q=[cos(ph/2) a(1)*sin(ph/2) a(2)*sin(ph/2) a(3)*sin(ph/2)];

t=rad2deg(t);
ph=rad2deg(ph);
end

== matlab function DinsatHW7/Dynamic Eq ==
  data: Inertia input size=[3 3]; omegaDot output size=3; omega input size=3; Torsion input size=3
function omegaDot = DynamicEq(Inertia,omega,Torsion)

omega=deg2rad(omega);

line1=Torsion(1)-omega(2)*(Inertia(3,1)*omega(1)+Inertia(3,2)*omega(2)+Inertia(3,3)*omega(3))+omega(3)*(Inertia(2,1)*omega(1)+Inertia(2,2)*omega(2)+Inertia(2,3)*omega(3));
line2=Torsion(2)-omega(3)*(Inertia(1,1)*omega(1)+Inertia(1,2)*omega(2)+Inertia(1,3)*omega(3))+omega(1)*(Inertia(3,1)*omega(1)+Inertia(3,2)*omega(2)+Inertia(3,3)*omega(3));
line3=Torsion(3)-omega(1)*(Inertia(2,1)*omega(1)+Inertia(2,2)*omega(2)+Inertia(2,3)*omega(3))+omega(2)*(Inertia(1,1)*omega(1)+Inertia(1,2)*omega(2)+Inertia(1,3)*omega(3));

omegaDot=Inertia\[line1;line2;line3];

omegaDot=rad2deg(omegaDot);

== matlab function DinsatHW7/GravityGrad ==
  data: r input size=[1 3]; Torsion output size=[1 3]; R_bodyorb input size=[3 3]; I input size=[3 3]
function Torsion = GravityGrad(r,R_bodyorb,I)
mu=3.986e5;
u=R_bodyorb\[0;0;1];
vec=cross(u,I*u);
Torsionn=3*mu/(norm(r)^3)*vec;
Torsion=Torsionn';

== matlab function DinsatHW7/MATLAB Function10 ==
  data: q_real input size=[1 4]; sigma output size=[1 3]; q_comm input size=[1 4]
function sigma = delq(q_real,q_comm)

q=q_comm;
qq=q_real;

qres=[q(1)*qq(1)+q(2)*qq(2)+q(3)*qq(3)+q(4)*qq(4);
    -q(2)*qq(1)+q(1)*qq(2)+q(4)*qq(3)-q(3)*qq(4);
    -q(3)*qq(1)-q(4)*qq(2)+q(1)*qq(3)+q(2)*qq(4);
    -q(4)*qq(1)+q(3)*qq(2)-q(2)*qq(3)+q(1)*qq(4)];

aa=qres(1,:)*2;
a=qres(2,:);
b=qres(3,:);
c=qres(4,:);

zz=[a,b,c];

sigma=aa*zz;

== matlab function DinsatHW7/MATLAB Function8 ==
  data: q_real input size=[1 4]; sigma output size=[1 3]; q_comm input size=[1 4]
function sigma = delq(q_real,q_comm)

q=q_comm;
qq=q_real;

qres=[q(1)*qq(1)+q(2)*qq(2)+q(3)*qq(3)+q(4)*qq(4);
    -q(2)*qq(1)+q(1)*qq(2)+q(4)*qq(3)-q(3)*qq(4);
    -q(3)*qq(1)-q(4)*qq(2)+q(1)*qq(3)+q(2)*qq(4);
    -q(4)*qq(1)+q(3)*qq(2)-q(2)*qq(3)+q(1)*qq(4)];

aa=qres(1,:)*2;
a=qres(2,:);
b=qres(3,:);
c=qres(4,:);

zz=[a,b,c];

sigma=aa*zz;

== matlab function DinsatHW7/MATLAB Function9 ==
  data: seq input; t input; q output size=[1 4]
function q=EulerAngles(seq,t)
t=deg2rad(t);

%% Rotation Matrix
%Rotasi pertama
i=[mod(seq(1)+1,3),mod(seq(1)+2,3)];
for j=1:2
    if i(j)==0
        i(j)=3;
    end
end
R_1=zeros(3,3);
R_1(i,i)=[cos(t(1)) sin(t(1));-sin(t(1)) cos(t(1))];
R_1(seq(1),seq(1))=1;

%Rotasi kedua
i=[mod(seq(2)+1,3),mod(seq(2)+2,3)];
for j=1:2
    if i(j)==0
        i(j)=3;
    end
end
R_2=zeros(3,3);
R_2(i,i)=[cos(t(2)) sin(t(2));-sin(t(2)) cos(t(2))];
R_2(seq(2),seq(2))=1;

%Rotasi ketiga
i=[mod(seq(3)+1,3),mod(seq(3)+2,3)];
for j=1:2
    if i(j)==0
        i(j)=3;
    end
end
R_3=zeros(3,3);
R_3(i,i)=[cos(t(3)) sin(t(3));-sin(t(3)) cos(t(3))];
R_3(seq(3),seq(3))=1;


R=R_3*R_2*R_1;
%% Euler axis and angle
%euler angle
ph=acos((trace(R)-1)/2);
if or(ph==pi,ph==0)
    a=0.5/sin(ph-1e-5)*([R(2,3)-R(3,2);R(3,1)-R(1,3);R(1,2)-R(2,1)]);
else
    a=0.5/sin(ph)*([R(2,3)-R(3,2);R(3,1)-R(1,3);R(1,2)-R(2,1)]);
end
%% quaternion
q=[cos(ph/2) a(1)*sin(ph/2) a(2)*sin(ph/2) a(3)*sin(ph/2)];

end

== matlab function DinsatHW7/MATLAB Function7 ==
  data: q_real input size=[1 4]; sigma output size=[1 3]; q_comm input size=[1 4]
function sigma = delq(q_real,q_comm)

q=q_comm;
qq=q_real;

qres=[q(1)*qq(1)+q(2)*qq(2)+q(3)*qq(3)+q(4)*qq(4);
    -q(2)*qq(1)+q(1)*qq(2)+q(4)*qq(3)-q(3)*qq(4);
    -q(3)*qq(1)-q(4)*qq(2)+q(1)*qq(3)+q(2)*qq(4);
    -q(4)*qq(1)+q(3)*qq(2)-q(2)*qq(3)+q(1)*qq(4)];

aa=qres(1,:)*2;
a=qres(2,:);
b=qres(3,:);
c=qres(4,:);

zz=[a,b,c];

sigma=aa*zz;

== matlab function DinsatHW7/MATLAB Function12 ==
  data: seq input; t input; q output size=[1 4]
function q=EulerAngles(seq,t)
t=deg2rad(t);

%% Rotation Matrix
%Rotasi pertama
i=[mod(seq(1)+1,3),mod(seq(1)+2,3)];
for j=1:2
    if i(j)==0
        i(j)=3;
    end
end
R_1=zeros(3,3);
R_1(i,i)=[cos(t(1)) sin(t(1));-sin(t(1)) cos(t(1))];
R_1(seq(1),seq(1))=1;

%Rotasi kedua
i=[mod(seq(2)+1,3),mod(seq(2)+2,3)];
for j=1:2
    if i(j)==0
        i(j)=3;
    end
end
R_2=zeros(3,3);
R_2(i,i)=[cos(t(2)) sin(t(2));-sin(t(2)) cos(t(2))];
R_2(seq(2),seq(2))=1;

%Rotasi ketiga
i=[mod(seq(3)+1,3),mod(seq(3)+2,3)];
for j=1:2
    if i(j)==0
        i(j)=3;
    end
end
R_3=zeros(3,3);
R_3(i,i)=[cos(t(3)) sin(t(3));-sin(t(3)) cos(t(3))];
R_3(seq(3),seq(3))=1;


R=[0,0,-1;0,1,0;1,0,0]*R_3*R_2*R_1;
%% Euler axis and angle
%euler angle
ph=acos((trace(R)-1)/2);
if or(ph==pi,ph==0)
    a=0.5/sin(ph-1e-5)*([R(2,3)-R(3,2);R(3,1)-R(1,3);R(1,2)-R(2,1)]);
else
    a=0.5/sin(ph)*([R(2,3)-R(3,2);R(3,1)-R(1,3);R(1,2)-R(2,1)]);
end
%% quaternion
q=[cos(ph/2) a(1)*sin(ph/2) a(2)*sin(ph/2) a(3)*sin(ph/2)];

end

== matlab function DinsatHW7/MATLAB Function13 ==
  data: u input; y output
function y = fcn(u)
if u(3)>0
    dec=asin(u(3)/norm(u));
else
    dec=-asin(abs(u(3)/norm(u)));
end
if u(2)>0
    RA=acos(u(1)/(norm(u)*cos(dec)));
else
    RA=-acos(u(1)/(norm(u)*cos(dec)));
end

y=rad2deg([RA,-dec,0]);

== matlab function DinsatHW7/MATLAB Function ==
  data: omega input; EulerAngleDot output size=[1 3]; seq input; EulerAngle input size=3
function EulerAngleDot= Omega2EulerAngleDot(omega,seq,EulerAngle)
EulerAngle=deg2rad(EulerAngle);
omega=deg2rad(omega);
if seq(1)==seq(3)
    det=sin(EulerAngle(2));
else
    det=cos(EulerAngle(2));
end
S_inverse=zeros(3,3);
S_inverse(3,seq(3))=1;
notseq=0;
for i=1:3
     if and(seq(1)~=i,seq(2)~=i)
         notseq=i;
     end
 end
 
if seq(1)==seq(3)
    if mod(seq(2)-seq(1),3)==1
        S_inverse(:,[seq(2) notseq])=[sin(EulerAngle(3)) cos(EulerAngle(3));
                                      cos(EulerAngle(3))*sin(EulerAngle(2)) -sin(EulerAngle(3))*sin(EulerAngle(2));
                                      -cos(EulerAngle(2))*sin(EulerAngle(3)) -cos(EulerAngle(2))*cos(EulerAngle(3))];
    else
        S_inverse(:,[seq(2) notseq])=[sin(EulerAngle(3)) -cos(EulerAngle(3));
                                      cos(EulerAngle(3))*sin(EulerAngle(2)) sin(EulerAngle(3))*sin(EulerAngle(2));
                                      -cos(EulerAngle(2))*sin(EulerAngle(3)) cos(EulerAngle(2))*cos(EulerAngle(3))];
    end
else
    if mod(seq(2)-seq(1),3)==1
        S_inverse(:,[seq(1) seq(2)])=[cos(EulerAngle(3)) -sin(EulerAngle(3));
                                      sin(EulerAngle(3))*cos(EulerAngle(2)) cos(EulerAngle(3))*cos(EulerAngle(2));
                                      -sin(EulerAngle(2))*cos(EulerAngle(3)) sin(EulerAngle(2))*sin(EulerAngle(3))];
    else
        S_inverse(:,[seq(1) seq(2)])=[cos(EulerAngle(3)) sin(EulerAngle(3));
                                      -sin(EulerAngle(3))*cos(EulerAngle(2)) cos(EulerAngle(3))*cos(EulerAngle(2));
                                      sin(EulerAngle(2))*cos(EulerAngle(3)) sin(EulerAngle(2))*sin(EulerAngle(3))];
    end
end
S_inverse=S_inverse/det;
EulerAngleDot=(S_inverse*omega)';
EulerAngleDot=rad2deg(EulerAngleDot);
end

== matlab function DinsatHW7/MATLAB Function2 ==
  data: u input; t output
function t = fcn(u)
t = rad2deg(atan2(sin(deg2rad(u)),cos(deg2rad(u))));

== matlab function DinsatHW7/Newton Gravity Equation/MATLAB Function3 ==
  data: r input size=[1 3]; a output size=[1 3]; mu input size=1
function a = GravForce(r,mu)
a=-mu/(norm(r)^3)*r;
end

== matlab function DinsatHW7/MATLAB Function3 ==
  data: v_init output size=[1 3]; r_init output size=[1 3]; sma input size=1; ecc input size=1; inc input size=1; node input size=1; aop input size=1; TA input size=1
function [v_init,r_init]=Keplerian2State(sma,ecc,inc,node,aop,TA)
inc=deg2rad(inc);
node=deg2rad(node);
aop=deg2rad(aop);
TA=deg2rad(TA);
mu=3.986004415e5;
if ecc~=1
    p=sma*(1-ecc^2);
else
    p=2*sma;
end
r_orb=[p*cos(TA)/(1+ecc*cos(TA));p*sin(TA)/(1+ecc*cos(TA));0];
v_orb=[-sqrt(mu/p)*sin(TA);sqrt(mu/p)*(ecc+cos(TA));0];

TRF=[cos(node)*cos(aop)-sin(node)*sin(aop)*cos(inc) -cos(node)*sin(aop)-sin(node)*cos(aop)*cos(inc) sin(node)*sin(inc);
    sin(node)*cos(aop)+cos(node)*sin(aop)*cos(inc) -sin(node)*sin(aop)+cos(node)*cos(aop)*cos(inc) -cos(node)*sin(inc);
    sin(aop)*sin(inc) cos(aop)*sin(inc) cos(inc)];

r=TRF*r_orb;
v=TRF*v_orb;
r_init=r';
v_init=v';
end

== matlab function DinsatHW7/MATLAB Function4 ==
  data: r input size=[1 3]; p output size=1; v input size=[1 3]; sma output size=1; ecc output size=1; inc output size=1; node output size=1; aop output size=1; TA output size=1
function [p,sma,ecc,inc,node,aop,TA]=State2Keplerian(r,v)
r=r';
v=v';
mu=3.986004415e5;
h=zeros(3,1);
n=zeros(3,1);
e=zeros(3,1);
h=cross(r,v);
n=cross([0;0;1],h);
e=((norm(v)^2-mu/norm(r))*r-(dot(r,v)*v))/mu;
ecc=norm(e);
xi=norm(v)^2/2-mu/norm(r);
inc=0;
TA=0;
if ecc~=1
    sma=-mu/(2*xi);
    p=sma*(1-ecc^2);
else
    p=norm(h)^2/mu;
    sma=inf;
end
inc=acos(h(3,1)/norm(h));
node=acos(n(1,1)/norm(n));
if n(2,1)<0
    node=2*pi-node;
end
aop=acos(dot(n,e)/(norm(n)*norm(e)));
if e(3,1)<0
    aop=2*pi-aop;
end
TA=acos(dot(e,r)/(norm(e)*norm(r)));
if dot(r,v)<0
    TA=2*pi-TA;
end
inc=rad2deg(inc);node=rad2deg(node);aop=rad2deg(aop);TA=rad2deg(TA);
end

== matlab function DinsatHW7/MATLAB Function5 ==
  data: seq input; t output; t input; R output size=[3 3]; a output size=[3 1]; ph output; q output size=[1 4]
function [t,R,a,ph,q]=EulerAngles(seq,t)
t=deg2rad(t);

%% Rotation Matrix
%Rotasi pertama
i=[mod(seq(1)+1,3),mod(seq(1)+2,3)];
for j=1:2
    if i(j)==0
        i(j)=3;
    end
end
R_1=zeros(3,3);
R_1(i,i)=[cos(t(1)) sin(t(1));-sin(t(1)) cos(t(1))];
R_1(seq(1),seq(1))=1;

%Rotasi kedua
i=[mod(seq(2)+1,3),mod(seq(2)+2,3)];
for j=1:2
    if i(j)==0
        i(j)=3;
    end
end
R_2=zeros(3,3);
R_2(i,i)=[cos(t(2)) sin(t(2));-sin(t(2)) cos(t(2))];
R_2(seq(2),seq(2))=1;

%Rotasi ketiga
i=[mod(seq(3)+1,3),mod(seq(3)+2,3)];
for j=1:2
    if i(j)==0
        i(j)=3;
    end
end
R_3=zeros(3,3);
R_3(i,i)=[cos(t(3)) sin(t(3));-sin(t(3)) cos(t(3))];
R_3(seq(3),seq(3))=1;

% perlu dikali rotasi dua kali lagi supaya benar koordinat orbitalnya
R=[1 0 0;0 0 -1;0 1 0]*[0 1 0;-1 0 0;0 0 1]*R_3*R_2*R_1;



%% menghitung di koordinat orbit ke inersial
seq=[1,2,3];
t1=[0,0];t2=[0,0];t3=[0,0];
notseq=0;
%% Euler angle
if seq(1,1)==seq(1,3)
    t2(1)=acos(R(seq(1),seq(3)));
    t2(2)=-1*t2(1);
    for i=1:3
        if and(seq(1)~=i,seq(2)~=i)
            notseq=i;
        end
    end
    if mod(seq(2)-seq(1),3)==2
    t1=atan2(R(seq(1),seq(2))./sin(t2),R(seq(1),notseq)./sin(t2));
    t3=atan2(R(seq(2),seq(1))./sin(t2),-R(notseq,seq(1))./sin(t2));
    else
    t1=atan2(R(seq(1),seq(2))./sin(t2),-R(seq(1),notseq)./sin(t2));   
    t3=atan2(R(seq(2),seq(1))./sin(t2),R(notseq,seq(1))./sin(t2));
    end
else
    if mod(seq(2)-seq(1),3)==2
    t2(1)=asin(-R(seq(3),seq(1)));
    t2(2)=pi-t2(1);
    t1=atan2(R(seq(3),seq(2))./cos(t2),R(seq(3),seq(3))./cos(t2));
    t3=atan2(R(seq(2),seq(1))./cos(t2),R(seq(1),seq(1))./cos(t2));
    else
    t2(1)=asin(R(seq(3),seq(1)));
    t2(2)=pi-t2(1);
    t1=atan2(-R(seq(3),seq(2))./cos(t2),R(seq(3),seq(3))./cos(t2));
    t3=atan2(-R(seq(2),seq(1))./cos(t2),R(seq(1),seq(1))./cos(t2));
    end   
end

%% Euler axis and angle
%euler angle
ph=acos((trace(R)-1)/2);
if or(ph==pi,ph==0)
    a=0.5/sin(ph-1e-5)*([R(2,3)-R(3,2);R(3,1)-R(1,3);R(1,2)-R(2,1)]);
else
    a=0.5/sin(ph)*([R(2,3)-R(3,2);R(3,1)-R(1,3);R(1,2)-R(2,1)]);
end
%% quaternion
q=[cos(ph/2) a(1,:)*sin(ph/2) a(2,:)*sin(ph/2) a(3,:)*sin(ph/2)];

t=[t1(1) t2(1) t3(1)];
t=rad2deg(t);
ph=rad2deg(ph);

end

== matlab function DinsatHW7/MATLAB Function6 ==
  data: R_BodyIner input size=[3 3]; RBodyOrbit output size=[3 3]; R_OrbitInertial input size=[3 3]
function RBodyOrbit = RotMatBodyInertial(R_BodyIner, R_OrbitInertial)
RBodyOrbit=R_BodyIner*inv(R_OrbitInertial);
end

== matlab function DinsatHW7/Attitude Body Orbit ==
  data: seq input size=[1 3]; t output size=[1 3]; R input size=[3 3]; R output; a output size=[3 1]; ph output; q output size=[1 4]
function [t,R,a,ph,q]=RotMatrix(seq,R)
t1=[0,0];t2=[0,0];t3=[0,0];
notseq=0;
%% Euler angle
if seq(1,1)==seq(1,3)
    t2(1)=acos(R(seq(1),seq(3)));
    t2(2)=-1*t2(1);
    for i=1:3
        if and(seq(1)~=i,seq(2)~=i)
            notseq=i;
        end
    end
    if mod(seq(2)-seq(1),3)==2
    t1=atan2(R(seq(1),seq(2))./sin(t2),R(seq(1),notseq)./sin(t2));
    t3=atan2(R(seq(2),seq(1))./sin(t2),-R(notseq,seq(1))./sin(t2));
    else
    t1=atan2(R(seq(1),seq(2))./sin(t2),-R(seq(1),notseq)./sin(t2));   
    t3=atan2(R(seq(2),seq(1))./sin(t2),R(notseq,seq(1))./sin(t2));
    end
else
    if mod(seq(2)-seq(1),3)==2
    t2(1)=asin(-R(seq(3),seq(1)));
    t2(2)=pi-t2(1);
    t1=atan2(R(seq(3),seq(2))./cos(t2),R(seq(3),seq(3))./cos(t2));
    t3=atan2(R(seq(2),seq(1))./cos(t2),R(seq(1),seq(1))./cos(t2));
    else
    t2(1)=asin(R(seq(3),seq(1)));
    t2(2)=pi-t2(1);
    t1=atan2(-R(seq(3),seq(2))./cos(t2),R(seq(3),seq(3))./cos(t2));
    t3=atan2(-R(seq(2),seq(1))./cos(t2),R(seq(1),seq(1))./cos(t2));
    end   
end

%% Euler axis and angle
%euler angle
ph=acos((trace(R)-1)/2);
if or(ph==pi,ph==0)
    a=0.5/sin(ph-1e-5)*([R(2,3)-R(3,2);R(3,1)-R(1,3);R(1,2)-R(2,1)]);
else
    a=0.5/sin(ph)*([R(2,3)-R(3,2);R(3,1)-R(1,3);R(1,2)-R(2,1)]);
end
%% quaternion
q=[cos(ph/2) a(1,:)*sin(ph/2) a(2,:)*sin(ph/2) a(3,:)*sin(ph/2)];

t=[t1(1) t2(1) t3(1)];
t=rad2deg(t);
ph=rad2deg(ph);

end
